simulink model "Amplitude_Modulation"  (R2025a)
settings: Solver=FixedStepDiscrete  StartTime=0.0  StopTime=0.000001  FixedStep=0.000000001  RelTol=1e-3
settings Model: Creator=anunn  LastModifiedBy=anunn

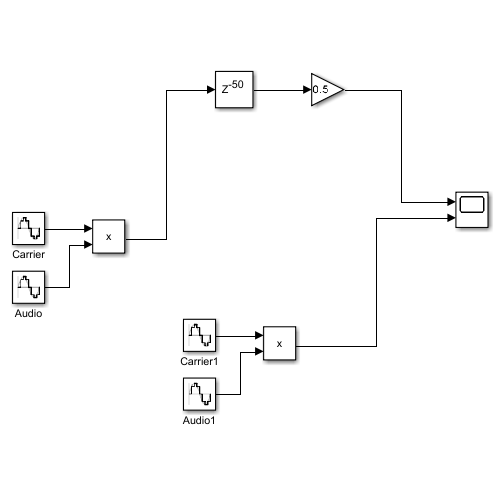
[thumbnail: Simulink's stored preview of the top-level diagram]
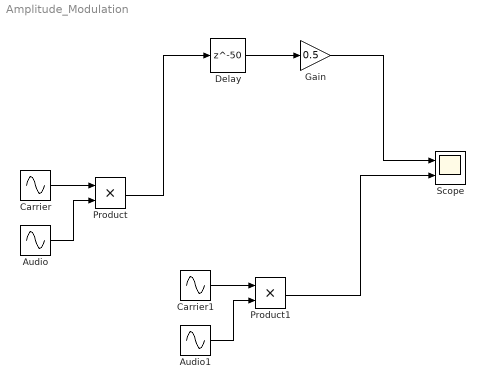
== system Amplitude_Modulation ==
  Audio : Sin  Frequency=6283185.3071796  SampleTime=0.000000001
  Audio1 : Sin  Frequency=6283185.3071796  SampleTime=0.000000001
  Carrier : Sin  Frequency=628318530.71796  SampleTime=0.000000001
  Carrier1 : Sin  Frequency=628318530.71796  SampleTime=0.000000001
  Delay : Delay  DelayLength=50
  Gain : Gain  Gain=0.5
  Product : Product
  Product1 : Product
  Scope : Scope  NumInputPorts=2
  wires:
  Carrier/1 -> Product/1
  Delay/1 -> Gain/1
  Gain/1 -> Scope/1
  Audio/1 -> Product/2
  Product/1 -> Delay/1
  Carrier1/1 -> Product1/1
  Product1/1 -> Scope/2
  Audio1/1 -> Product1/2
